simulink model "gm_overflow_and_saturation"  (R2016b)
settings: Solver=VariableStepAuto  StartTime=0.0  StopTime=10  RelTol=1e-3
settings Model: Creator=Arthur  LastModifiedBy=Arthur
settings OptimizationCC: BlockReduction=off  ConditionallyExecuteInputs=off
settings DebuggingCC: InheritedTsInSrcMsg=none

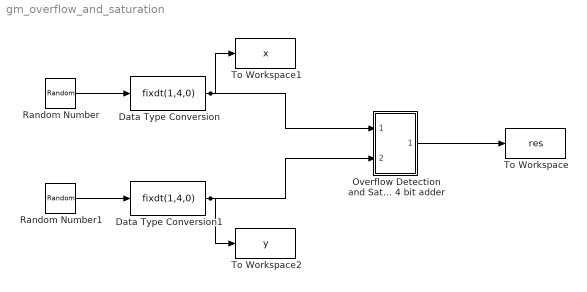
== system gm_overflow_and_saturation ==
  Data Type Conversion : DataTypeConversion  OutDataTypeStr=fixdt(1,4,0)
  Data Type Conversion1 : DataTypeConversion  OutDataTypeStr=fixdt(1,4,0)
  Overflow Detection and Saturation 4 bit adder : Subsystem
  Random Number : RandomNumber  Variance=10  SampleTime=1
  Random Number1 : RandomNumber  Variance=20  Seed=1  SampleTime=1
  To Workspace : ToWorkspace  VariableName=res  SampleTime=-1
  To Workspace1 : ToWorkspace  VariableName=x  SampleTime=-1
  To Workspace2 : ToWorkspace  VariableName=y  SampleTime=-1
  wires:
  Overflow Detection and Saturation 4 bit adder/1(Out1) -> To Workspace/1
  Random Number1/1 -> Data Type Conversion1/1
  Random Number/1 -> Data Type Conversion/1
  Data Type Conversion1/1 -> To Workspace2/1, Overflow Detection and Saturation 4 bit adder/2(In2)
  Data Type Conversion/1 -> To Workspace1/1, Overflow Detection and Saturation 4 bit adder/1(In1)

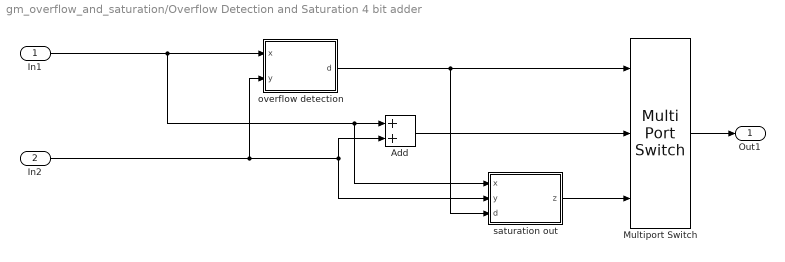
== system gm_overflow_and_saturation/Overflow Detection and Saturation 4 bit adder ==
  In1 : Inport
  In2 : Inport  Port=2
  Add : Sum  OutDataTypeStr=fixdt(1,4,0)
  Multiport Switch : MultiPortSwitch  DataPortOrder=Zero-based contiguous  Inputs=2  OutDataTypeStr=fixdt(1,4,0)
  overflow detection : MATLAB Function  TreatAsAtomicUnit=on
  saturation out : MATLAB Function  TreatAsAtomicUnit=on
  Out1 : Outport
  wires:
  overflow detection/1(d) -> Multiport Switch/1, saturation out/3(d)
  Add/1 -> Multiport Switch/2
  saturation out/1(z) -> Multiport Switch/3
  Multiport Switch/1 -> Out1/1
  In2/1 -> saturation out/2(y), Add/2, overflow detection/2(y)
  In1/1 -> Add/1, saturation out/1(x), overflow detection/1(x)

== matlab function gm_overflow_and_saturation/Overflow Detection and Saturation 4 bit adder/saturation out ==
  data: x input; z output; y input; d input
function z = fcn(x,y,d)

s1 = bitget(x,4);
s2 = bitget(y,4);

if (d == 1)
    if(bitand(s1,s2))
        z = fi(-8,1,4,0);
    else
        z = fi(7,1,4,0);
    end
else
    z = x;      % this path is irrelevant
end

== matlab function gm_overflow_and_saturation/Overflow Detection and Saturation 4 bit adder/overflow detection ==
  data: d output; x input; y input
function d = fcn(x,y)

x0 = bitget(x,1);
x1 = bitget(x,2);
x2 = bitget(x,3);
x3 = bitget(x,4);

y0 = bitget(y,1);
y1 = bitget(y,2);
y2 = bitget(y,3);
y3 = bitget(y,4);

c1 = bitand(x0, y0);

t1 = bitand(x1,y1);
t2 = bitand(bitor(x1,y1),c1);
c2 = bitor(t1,t2);

t1 = bitand(x2,y2);
t2 = bitand(bitor(x2,y2),c2);
c3 = bitor(t1,t2);

t1 = bitand(x3,y3);
t2 = bitand(bitor(x3,y3),c3);
c4 = bitor(t1,t2);

d = bitxor(c4, c3);
